simulink model "hyperloop_arc_org"  (Simulink 10.0)
settings: Solver=ode45  StartTime=0.0  StopTime=inf  FixedStep=0.01  RelTol=1e-3  EnableMultiTasking=on
StopFcn:
  | stopFcn_hyperloop_arc
libraries: Chassis_Alpha x1, Chassis_Alpha_sm x1, Chassis_Alpha_sm_s3d x1, Compressor_Alpha x1, Compressor_Defaults x1, simulink x1, Power_Alpha x1, Prop_Alpha x1, Tube_Alpha x1, Tube_Alpha_sf x1
Description:
  | Model of the hyperloop transportation concept put forward in the Alpha proposal
  | (hyperloop_alpha-20130812.pdf) from SpaceX/Tesla. Model is intended for open
  | contribution.
  | 
  | Copyright 2013-2014 The MathWorks, Inc.
settings Model: Creator=mbrauer  LastModifiedBy=annonymous
settings DataIOCC: Decimation=10  LimitDataPoints=on  InspectSignalLogs=on
settings OptimizationCC: BlockReduction=off  DefaultParameterBehavior=Inlined  BufferReuse=off
settings DebuggingCC: AlgebraicLoopMsg=none  ParameterPrecisionLossMsg=none  UnconnectedInputMsg=none  UnconnectedOutputMsg=none  UnconnectedLineMsg=none  SFUnusedDataAndEventsDiag=none
settings GRTTargetCC: GeneratePreprocessorConditionals=Disable all  CombineOutputUpdateFcns=on  GRTInterface=off
settings ConfigComp: CovExternalEMLEnable=off  CovSFcnEnable=off
settings SimscapeCC: SimscapeNormalizeSystem=off
settings ConfigurationSet: Description=SimMechanics 2G
settings ExplorerConfigSet: InternalSimMechanicsExplorerSettings="<ExplorerConfiguration><canonicalview>default</canonicalview><AnimationSetting><BasePlaybackSpeed>1.0</BasePlaybackSpeed><PlaybackSpeedFactor>1.0</PlaybackSpeedFactor></AnimationSetting><TilePanel><TileInfo><Tiles Columns=\"1\" Count=\"1\" Rows=\"1\"><Column Left=\"2\" Weight=\"1\"/><Column Left=\"884\"/><Row Top=\"2\" Weight=\"1\"/><Row Top=\"811\"/><Tile Height=\"1\" Width=\"1\" X=\"0\" Y=\"0\"/></Tiles></TileInfo><SceneInfo><SceneViewer><BGColor><R>0.60000002384185791</R><G>0.60000002384185791</G><B>0.60000002384185791</B></BGColor><Camera><Position><X>0</X><Y>0</Y><Z>3.2527065277099609</Z></Position><Center><X>0</X><Y>0</Y><Z>0</Z></Center><Up><X>0</X><Y>1</Y><Z>-0</Z></Up><Left>-1.2074999749660493</Left><Right>1.2074999749660493</Right><Bottom>-1.2074999749660493</Bottom><Top>1.2074999749660493</Top></Camera></SceneViewer></SceneInfo></TilePanel></ExplorerConfiguration>"

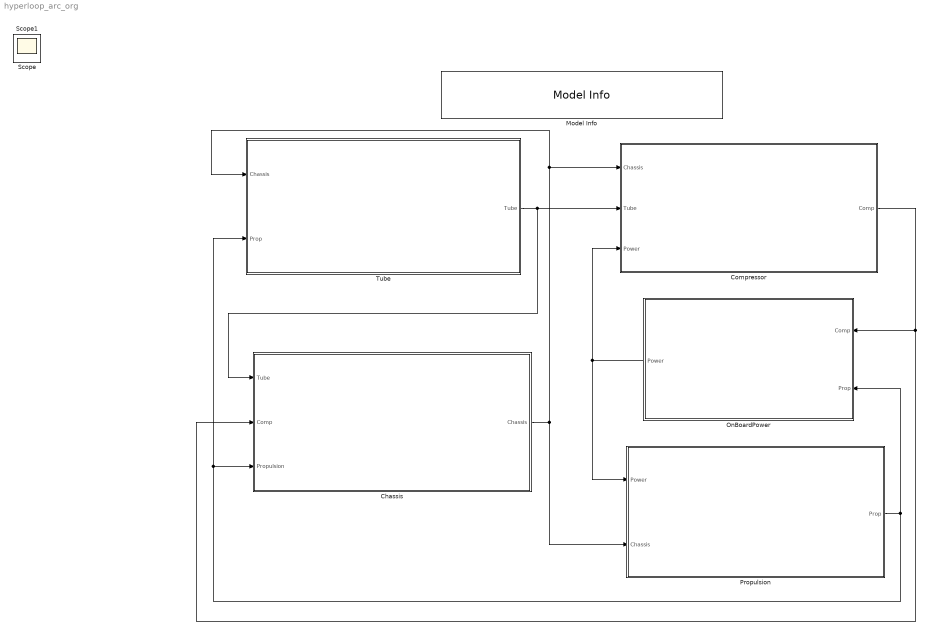
== system hyperloop_arc_org ==
  Chassis : Subsystem  Variant=on
      mask Display: image('Chassis.png',[110 10 200 150])
  Compressor : Subsystem  Variant=on
      mask Display: image('Compressor.png',[90 10 200 135])
  Model Info : simulink/Model-Wide Utilities/Model Info  Frame=on  DisplayStringWithTags=%<Description>  HorizontalTextAlignment=Center  LeftAlignmentValue=0.5
  OnBoardPower : Subsystem  Variant=on
      mask Display: image('OnBoardPower.png',[70 20 170 120])
  Propulsion : Subsystem  Variant=on
      mask Display: image('Propulsion.png',[90 10 200 155])
  Tube : Subsystem  Variant=on
      mask Display: image('Tube.png',[0.2 0.05 0.6 0.75])
  Scope : Scope
  Scope1 : Scope
  wires:
  Propulsion/1(Prop) -> OnBoardPower/2(Prop), Tube/2(Prop), Chassis/3(Propulsion)
  Compressor/1(Comp) -> Chassis/2(Comp), OnBoardPower/1(Comp)
  OnBoardPower/1(Power) -> Propulsion/1(Power), Compressor/3(Power)
  Tube/1(Tube) -> Chassis/1("Tube "), Compressor/2(Tube)
  Chassis/1(Chassis) -> Tube/1(Chassis), Compressor/1(Chassis), Propulsion/2(Chassis)

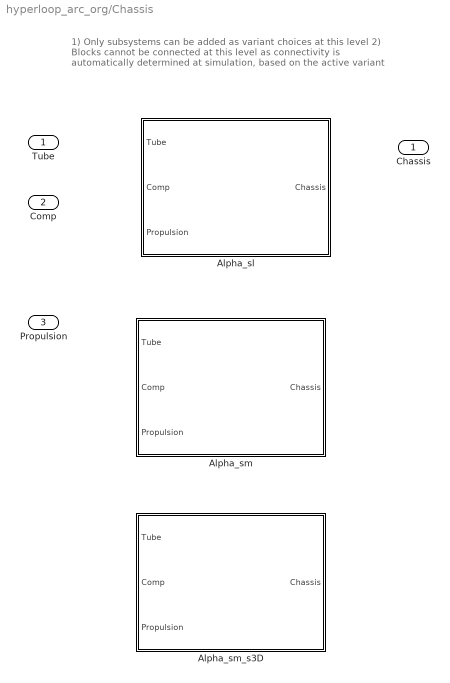
== system hyperloop_arc_org/Chassis ==
  note: 1) Only subsystems can be added as variant choices at this level
      | 2) Blocks cannot be connected at this level as connectivity is
      | automatically determined at simulation, based on the active variant
  "Tube " : Inport
  Comp : Inport  Port=2
  Propulsion : Inport  Port=3
  Alpha_sl : Subsystem  VariantControl=VAR_Chassis==varChassis.Alpha
  Alpha_sm : Subsystem  VariantControl=VAR_Chassis==varChassis.Alpha_sm
  Alpha_sm_s3D : Subsystem  VariantControl=VAR_Chassis==varChassis.Alpha_sm_s3D
  Chassis : Outport

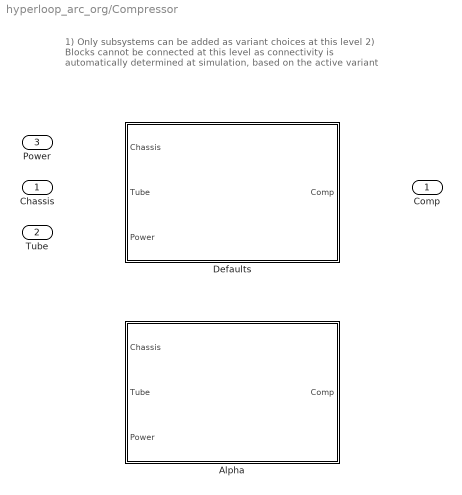
== system hyperloop_arc_org/Compressor ==
  note: 1) Only subsystems can be added as variant choices at this level
      | 2) Blocks cannot be connected at this level as connectivity is
      | automatically determined at simulation, based on the active variant
  Chassis : Inport
  Tube : Inport  Port=2
  Power : Inport  Port=3
  Alpha : Subsystem  VariantControl=VAR_COMP==varComp.Alpha
  Defaults : Subsystem  VariantControl=VAR_COMP==varComp.Defaults
  Comp : Outport

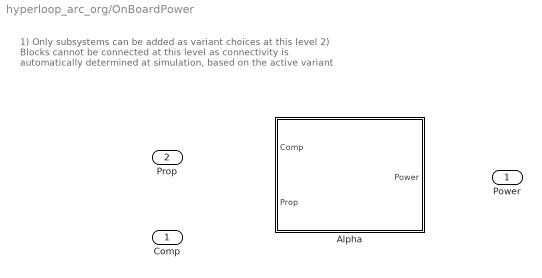
== system hyperloop_arc_org/OnBoardPower ==
  note: 1) Only subsystems can be added as variant choices at this level
      | 2) Blocks cannot be connected at this level as connectivity is
      | automatically determined at simulation, based on the active variant
  Comp : Inport
  Prop : Inport  Port=2
  Alpha : Subsystem  VariantControl=VAR_POWER==varPower.Alpha
  Power : Outport

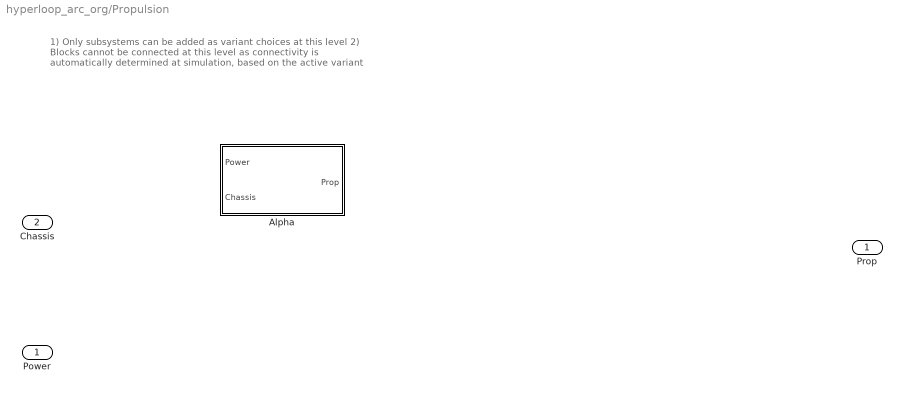
== system hyperloop_arc_org/Propulsion ==
  note: 1) Only subsystems can be added as variant choices at this level
      | 2) Blocks cannot be connected at this level as connectivity is
      | automatically determined at simulation, based on the active variant
  Power : Inport
  Chassis : Inport  Port=2
  Alpha : Subsystem  VariantControl=VAR_PROP==varProp.Alpha
  Prop : Outport

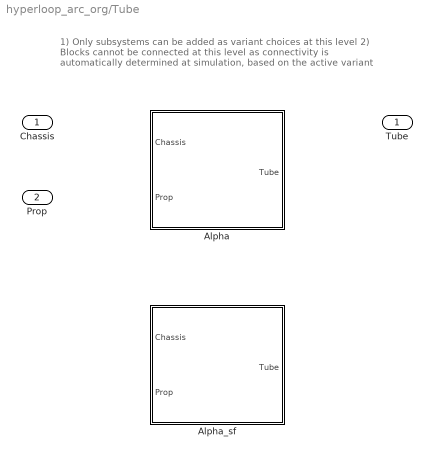
== system hyperloop_arc_org/Tube ==
  note: 1) Only subsystems can be added as variant choices at this level
      | 2) Blocks cannot be connected at this level as connectivity is
      | automatically determined at simulation, based on the active variant
  Chassis : Inport
  Prop : Inport  Port=2
  Alpha : Subsystem  VariantControl=VAR_TUBE == varTube.Alpha
  Alpha_sf : Subsystem  VariantControl=VAR_TUBE == varTube.Alpha_sf
  Tube : Outport

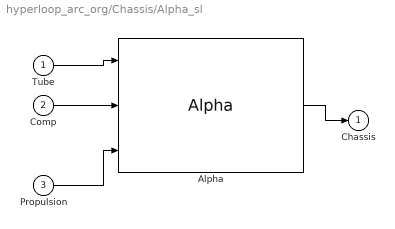
== system hyperloop_arc_org/Chassis/Alpha_sl ==
  "Tube " : Inport
  Comp : Inport  Port=2
  Propulsion : Inport  Port=3
  Alpha : Chassis_Alpha/Alpha
  Chassis : Outport
  wires:
  Propulsion/1 -> Alpha/3
  Comp/1 -> Alpha/2
  "Tube "/1 -> Alpha/1
  Alpha/1 -> Chassis/1

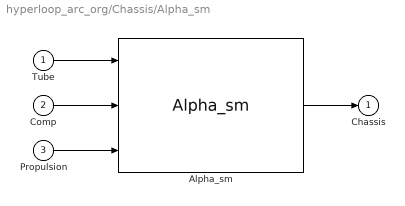
== system hyperloop_arc_org/Chassis/Alpha_sm ==
  "Tube " : Inport
  Comp : Inport  Port=2
  Propulsion : Inport  Port=3
  Alpha_sm : Chassis_Alpha_sm/Alpha_sm
  Chassis : Outport
  wires:
  Propulsion/1 -> Alpha_sm/3
  Comp/1 -> Alpha_sm/2
  "Tube "/1 -> Alpha_sm/1
  Alpha_sm/1 -> Chassis/1

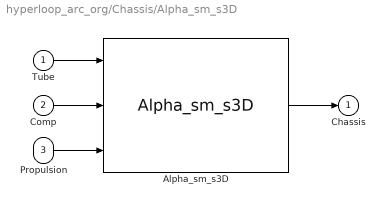
== system hyperloop_arc_org/Chassis/Alpha_sm_s3D ==
  "Tube " : Inport
  Comp : Inport  Port=2
  Propulsion : Inport  Port=3
  Alpha_sm_s3D : Chassis_Alpha_sm_s3d/Alpha_sm_s3D
  Chassis : Outport
  wires:
  "Tube "/1 -> Alpha_sm_s3D/1
  Comp/1 -> Alpha_sm_s3D/2
  Propulsion/1 -> Alpha_sm_s3D/3
  Alpha_sm_s3D/1 -> Chassis/1

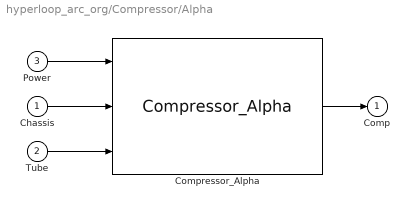
== system hyperloop_arc_org/Compressor/Alpha ==
  Chassis : Inport
  Tube : Inport  Port=2
  Power : Inport  Port=3
  Compressor_Alpha : Compressor_Alpha/Compressor_Alpha
  Comp : Outport
  wires:
  Power/1 -> Compressor_Alpha/1
  Chassis/1 -> Compressor_Alpha/2
  Tube/1 -> Compressor_Alpha/3
  Compressor_Alpha/1 -> Comp/1

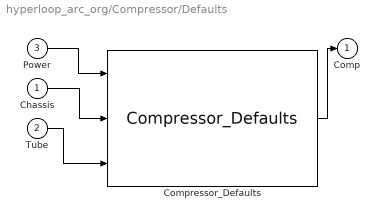
== system hyperloop_arc_org/Compressor/Defaults ==
  Chassis : Inport
  Tube : Inport  Port=2
  Power : Inport  Port=3
  Compressor_Defaults : Compressor_Defaults/Compressor_Defaults  VariantControl=VAR_Compressor_Defaults
  Comp : Outport
  wires:
  Power/1 -> Compressor_Defaults/1
  Chassis/1 -> Compressor_Defaults/2
  Tube/1 -> Compressor_Defaults/3
  Compressor_Defaults/1 -> Comp/1

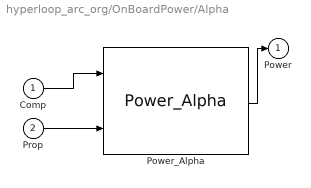
== system hyperloop_arc_org/OnBoardPower/Alpha ==
  Comp : Inport
  Prop : Inport  Port=2
  Power_Alpha : Power_Alpha/Power_Alpha
  Power : Outport
  wires:
  Comp/1 -> Power_Alpha/1
  Prop/1 -> Power_Alpha/2
  Power_Alpha/1 -> Power/1

== system hyperloop_arc_org/Propulsion/Alpha ==
  Power : Inport
  Chassis : Inport  Port=2
  Prop_Alpha : Prop_Alpha/Prop_Alpha
  Prop : Outport
  wires:
  Prop_Alpha/1 -> Prop/1
  Chassis/1 -> Prop_Alpha/1
  Power/1 -> Prop_Alpha/2

== system hyperloop_arc_org/Tube/Alpha ==
  Chassis : Inport
  Prop : Inport  Port=2
  Tube_Alpha : Tube_Alpha/Tube_Alpha  VariantControl=VAR_Tube_Alpha
  Tube : Outport
  wires:
  Chassis/1 -> Tube_Alpha/1
  Prop/1 -> Tube_Alpha/2
  Tube_Alpha/1 -> Tube/1

== system hyperloop_arc_org/Tube/Alpha_sf ==
  Chassis : Inport
  Prop : Inport  Port=2
  Tube_Alpha_sf : Tube_Alpha_sf/Tube_Alpha_sf  VariantControl=VAR_Tube_Alpha
  Tube : Outport
  wires:
  Chassis/1 -> Tube_Alpha_sf/1
  Prop/1 -> Tube_Alpha_sf/2
  Tube_Alpha_sf/1 -> Tube/1
